simulink model "RealLifeTrainModel"  (R2024a)
settings: Solver=ode1  StartTime=0.0  StopTime=Inf  FixedStep=0.001  RelTol=1e-3
PostLoadFcn:
  | , if any(exist('dsrtsu_mdlpostloadfcn', 'file') ~= 0), dsrtsu_mdlpostloadfcn('Execute', bdroot); end,
InitFcn:
  | , if any(exist('rtifpga_mdlclblib', 'file') ~= 0), rtifpga_mdlclblib('Init', bdroot); end,
undefined symbols (not defined in the file): DiscIntNeverNeededParam
libraries: deeplib x29, svdutilitieslib x28, simulink x8, eeGeneralControl x8, rti1202lib_adc_class1 x6, rti1202serlib x5, spsEdgeDetectorLib x5, rtiemclib x2, rti1202lib_dac_class1 x1
(part 8 of 8)

== matlab function RealLifeTrainModel/ContractionMetricFilterSystem1/MATLAB Function ==
  data: x input; u_filtered output; ref input; u_nom input; dt input; task_dim input; row_major input; td_is_zero_based input; eps_pd input; use_A_transpose input; lambda_val input; last_ixv input; flag_start input; Kp input; Ki input; ref_denorm input; Dref_denorm input; integral_erro input; cert_val output; is_active output; a_val output; b_val output; du_out output; M_curr_out output; Mdot_out output; erro output; u_nom_teste output; A_m output; B_m output; K_m output; k1 input; k2 input; k3 input; dkp input; dki input; controller input
function [u_filtered, cert_val, is_active, a_val, b_val, du_out, M_curr_out, Mdot_out,erro,u_nom_teste,A_m,B_m,K_m] = ...
    qp_filter_projected_deltaU_getM( ...
        x, ref, u_nom, ...
        dt, task_dim, ...
        row_major, td_is_zero_based, eps_pd, use_A_transpose, lambda_val, ...
        last_ixv, flag_start, Kp, Ki, ref_denorm, Dref_denorm,integral_erro,k1,k2,k3,dkp,dki,controller) %#codegen

max_Fload =  569.629505294963
min_Fload = -610.339671010468

% Closed-form QP:  min 0.5*||Δu||^2  s.t. a'*Δu <= b,   u_filt = u_nom + Δu
% Uses your get_M(x) to build M(x) internally (no M_* inputs).
% A,B from FD on get_model([x;u]), K from FD on your policy(...).

% -------- defaults / casts (codegen-safe) --------
if nargin < 6  || isempty(row_major),        row_major        = true;  end %#ok<NASGU> % kept for API compat; get_M already fixes orientation
if nargin < 7  || isempty(td_is_zero_based), td_is_zero_based = true;  end
if nargin < 8  || isempty(eps_pd),           eps_pd           = single(1e-3); end
if nargin < 9  || isempty(use_A_transpose),  use_A_transpose  = false; end

tdZeroBased = (td_is_zero_based ~= 0);
useAT       = (use_A_transpose  ~= 0);

dt          = cast(dt,          'single');
eps_pd      = cast(eps_pd,      'single');
lambda_val  = cast(lambda_val,  'single');
Kp          = cast(Kp,          'single');
Ki          = cast(Ki,          'single');
ref_denorm  = cast(ref_denorm,  'single');
Dref_denorm = cast(Dref_denorm, 'single');
last_ixv    = cast(last_ixv,    'single');
flag_start  = cast(flag_start,  'single');

% -------- sizes / shapes --------
n   = int32(8);                 % state dim
m   = int32(1);                 % scalar control
x_m = reshape(x, [], 1);        % (n x 1), normalized [0,1]

% -------- Metric from your network --------
M_curr = cast(get_M(x_m), 'single');    % (8x8) SPD already
M_curr_out = M_curr;                    % expose for debug

% -------- Compute Mdot --------
persistent have_prev M_prev
if isempty(have_prev)
    have_prev = false;
    M_prev    = zeros(8,8,'single');
end

if flag_start ~= 0
    % reset at episode start
    have_prev = false;
end


M_dot = (M_curr - M_prev) ./ dt;    % time FD


% update persistent for next call
M_prev    = M_curr;
have_prev = true;

Mdot_out = M_dot;    % expose for debug

%policy(normdata,last_ixv,flag_start,ref_denorm,Kp,Ki,Dref_denorm,integral)
u_nom_teste = 2*policy_nominal_(x_m,ref,last_ixv,flag_start,Kp,Ki,ref_denorm,Dref_denorm,integral_erro,dkp,dki,controller) - 1

% -------- Linearize model: A = ∂f/∂x, B = ∂f/∂u --------
[A_m, B_m] = linearize_model_fd_(x_m, u_nom, n);

% -------- K from your policy (FD) --------

K_m = policy_jacobian_fd_(x_m, ref, last_ixv, flag_start, Kp, Ki, ref_denorm, Dref_denorm, n,integral_erro,dkp,dki,controller); % (1 x n)

% -------- ABK (+ optional Aᵀ) --------
A_use = A_m; if useAT, A_use = A_m.'; end
ABK   = A_use + B_m * K_m;     % (n x n)

% -------- Contraction matrix --------
symPart = M_curr * ABK;
symPart = symPart + symPart.'; 
C = M_dot + symPart + (2 * lambda_val) * M_curr;

% -------- contracting direction v --------
td = int32(task_dim); if tdZeroBased, td = td + 1; end
td = max(1, min(td, n));
v = zeros(n,1,'single');
v(td,1) = cast(x_m(td,1) - cast(ref,'like',x_m), 'single');

% -------- certificate & halfspace --------
cert_val = cast(v' * C * v, 'like', u_nom);      % scalar
a_row    = 2 * (v' * (M_curr * B_m));            % (1 x m)
e = ref - x(3)
b_val    = cast(-(v' * C * v), 'like', u_nom) - (k2 + k3*abs(e));   % scalar

% -------- closed-form projection in Δu-space --------
a_col  = cast(a_row.', 'like', u_nom);           % (m x 1)
anorm2 = max(cast(1e-12, 'like', u_nom), sum(a_col .* a_col));

if b_val >= 0
    du = zeros(m, 1, 'like', u_nom); active = 0;
else
    du = (b_val / anorm2) * a_col;   active = 1;
end

% elementwise clip Δu
du = min(max(du, -eps_pd), eps_pd);

u_filtered = u_nom + du + k1*(e);
is_active  = double(active);
a_val      = a_col;
du_out     = du;

force = x(3)*(max_Fload - min_Fload) + min_Fload

erro = ref_denorm - force
end

% ====================== helpers (codegen-safe) ======================

function y = clip01_(z)
% clamp to [0,1] (single, vector/scalar)
y = min(max(cast(z,'single'), cast(0,'single')), cast(1,'single'));
end

function [A_m, B_m] = linearize_model_fd_(x, u, n)
% Central FD on your ONNX-backed model get_model([x;u])
x = cast(x, 'single'); u = cast(u, 'single');
A_m = zeros(n, n, 'single');
B_m = zeros(n, 1, 'single');

eps_x = cast(1e-4, 'single');
eps_u = cast(1e-3, 'single');

xm = clip01_(x);
f = f_model_(x, u);

% A: ∂f/∂x
for i = 1:n
    dx = zeros(n,1,'single'); dx(i) = eps_x;
    xp = (x + dx);

    fp = f_model_(xp, u);

    A_m(:, i) = (fp - f) ./ (eps_x);
end

% B: ∂f/∂u
up = (u + eps_u);
ul = (u - eps_u);
xm = clip01_(x);
fp = f_model_(x, up);
fl = f_model_(x, ul);

B_m(:, 1) = (fp - f) ./ (eps_u);
end

function f = f_model_(x, u)
% Evaluate learned dynamics at (x,u); get_model expects 9x1 input [x; u]
xu = [cast(x,'single'); cast(u,'single')];
f  = cast(get_model(xu), 'single');   % (8x1)
end

function K = policy_jacobian_fd_(x, ref, last_ixv, flag_start, Kp, Ki, ref_denorm, Dref_denorm, n,integral,dkp,dki,controller)
% Central FD of your policy π(x, ref) using your provided function
K = zeros(1, n, 'single');
eps_x = cast(1e-3, 'single');
x_ = (x);
u = policy_nominal_(x_, ref, last_ixv, flag_start, Kp, Ki, ref_denorm, Dref_denorm,integral,dkp,dki,controller);

for i = 1:n
    dx = zeros(n,1,'single'); dx(i) = eps_x;
    xp = (x + dx);

    up = policy_nominal_(xp, ref, last_ixv, flag_start, Kp, Ki, ref_denorm, Dref_denorm,integral,dkp,dki,controller);

    K(1,i) = (up - u) ./ (eps_x);
end
end

function u = policy_nominal_(x, ref, last_ixv, flag_start, Kp, Ki, ref_denorm, Dref_denorm,integral,dkp,dki,controller)
% Thin wrapper to your policy(normdata,last_ixv,flag_start,ref_denorm,Kp,Ki,Dref_denorm)
normdata = [cast(x,'single'); cast(ref,'single')];  % 9x1, normalized
u = cast(policy(normdata, last_ixv, flag_start, ref_denorm, Kp, Ki, Dref_denorm,integral,dkp,dki,controller), 'single');
end


function y = get_model(x)
%#codegen
% x: 9x1 normalized in [0,1]
% y: 8x1 single, normalized to [0,1]
% y = y1 + (y2.^2) * u_scalar, then re-scale to [0,1]

% ---- normalize / split inputs ----
x_single = single(x(:));           % 9x1
x_scaled = 2*x_single - 1;         % [-1, 1]
feat     = x_scaled(1:8);          % 8x1
u_scalar = x_scaled(9);            % scalar

% ---- two pure-C forwards using saved weights ----
y1 = model_forward_m1(x_scaled);       % 8x1


% ---- combine and clamp ----

y  = 0.5 * y1 + 0.5;                % back to [0,1]
end


function M = get_M(x)
%#codegen
% x: 8x1 normalized in [0,1]
% M: 8x8 SPD single

x8  = single(x(:));                % 8x1

% metric net: 2-FC (64 outputs) → reshape to 8x8
v64 = metric_forward_2fc(x8);      % 64x1

n    = int32(8);
Mraw = reshape(v64, [n, n]).';                          % row-major → col-major
M    = (Mraw.' * Mraw) + single(1e-3) * eye(n,'single'); % SPD
end


% ==================== helpers (pure C, RTI-safe) ====================

function y = model_forward_m1(x8)
%#codegen
% 3-FC with ReLU after first two; outputs 8x1
persistent W1 b1 W2 b2 W3 b3 init
if isempty(init)
    S  = coder.load(coder.const('C:\Users\ic2d\Documents\GitHub\dSpace_Controllers_legged\model_smaller_weights.mat'));
    W1 = single(S.W1);  b1 = single(S.b1);   % [64x8],  [64x1]
    W2 = single(S.W2);  b2 = single(S.b2);   % [64x64], [64x1]
    W3 = single(S.W3);  b3 = single(S.b3);   % [8x64],  [8x1]
    init = true;
end
x8 = single(x8(:));
z1 = W1 * x8 + b1;   a1 = max(z1, single(0));   % ReLU
z2 = W2 * a1 + b2;   a2 = max(z2, single(0));   % ReLU
y  = W3 * a2 + b3;                              % 8x1
end

function y = model_forward_m2(x8)
%#codegen
% 3-FC with ReLU after first two; outputs 8x1
persistent W1 b1 W2 b2 W3 b3 init
if isempty(init)
    S  = coder.load(coder.const('C:\Users\ic2d\Documents\GitHub\dSpace_Controllers_legged\model_2_weights.mat'));
    W1 = single(S.W1);  b1 = single(S.b1);   % [64x8],  [64x1]
    W2 = single(S.W2);  b2 = single(S.b2);   % [64x64], [64x1]
    W3 = single(S.W3);  b3 = single(S.b3);   % [8x64],  [8x1]
    init = true;
end
x8 = single(x8(:));
z1 = W1 * x8 + b1;   a1 = max(z1, single(0));   % ReLU
z2 = W2 * a1 + b2;   a2 = max(z2, single(0));   % ReLU
y  = W3 * a2 + b3;                              % 8x1
end

function y64 = metric_forward_2fc(x8)
%#codegen
% 2-FC with ReLU after first; outputs 64x1
persistent W1 b1 W2 b2 init
if isempty(init)
    S  = coder.load(coder.const('C:\Users\ic2d\Documents\GitHub\dSpace_Controllers_legged\metric_new_weights.mat'));
    W1 = single(S.W1);  b1 = single(S.b1);   % [64x8],  [64x1]
    W2 = single(S.W2);  b2 = single(S.b2);   % [64x64], [64x1]
    init = true;
end
x8  = single(x8(:));
z1  = W1 * x8 + b1;                 % [64x1]
a1  = max(z1, single(0));           % ReLU
y64 = W2 * a1 + b2;                 % [64x1]
end


function y = policy(normdata,last_ixv,flag_start,ref_denorm,Kp,Ki,Dref_denorm,integral,dkp,dki,controller)

data = denorm(normdata)

y = FL(last_ixv,flag_start,data, Kp,Ki,Dref_denorm,ref_denorm,integral,dkp,dki,controller);

end


function y = denorm(u)
    max_Fload =  569.629505294963
    min_Fload = -610.339671010468
    
    max_Fhyd = 729.261146885585
    min_Fhyd = -777.489547410502
    
    max_DFload = 123011.265014651
    min_DFload = -142353.177843906
    
    max_DFhyd = 219994.429294316
    min_DFhyd = -270882.694509076
    
    max_Pa = 12037835.3221229
    min_Pa = 1849925.22965178
    
    max_Pb = 14831789.6053956
    min_Pb = 2808786.27887814
    
    max_x = 0.082368752
    min_x = 0.01990812
    
    max_Dx = 0.682789396628826
    min_Dx = -0.578996654196926
    
    out = [1,1,1,1,1,1,1,1,1]
    
    out(1) = (u(1))*(max_Fhyd - min_Fhyd) + min_Fhyd;
    
    out(2) = (u(2))*(max_DFhyd - min_DFhyd) + min_DFhyd;
    
    out(3) = (u(3))*(max_Fload - min_Fload) + min_Fload;
    
    out(4) = (u(4))*(max_DFload - min_DFload) + min_DFload;
    
    out(5) = (u(5))*(max_Pa - min_Pa) + min_Pa;
    
    out(6) = (u(6))*(max_Pb - min_Pb) + min_Pb;
    
    out(7) = (u(7))*(max_x - min_x) + min_x;
    
    out(8) = (u(8))*(max_Dx - min_Dx) + min_Dx;
    
    out(9) = (u(9))*(max_Fload - min_Fload) + min_Fload;
    
    
    y = out;
end

function y = FL(ixv,flag_start,data_denorm,Kp,Ki,Dref_denorm,Ref_denorm,integral,dkp,dki,controller)
    Pn = 7000000
    Qn = 10/60000
    Un = 0.05
    Be = 1.31E+9
    c1 = 0.8
    c2 = 1
    alfa = 0.609
    Vpl = 0.00121
    Ps = 16000000
    Pt = 0
    L_cyl = 0.08
    Aa = 0.000201
    
    if flag_start == 1
        data = data_denorm
        Pa = data(5)
        Pb = data(6)
        xp = data(7)
        xpd = data(8)
    
        Kv = Qn/(Un*sqrt(Pn/2));
        
        Va = Vpl + Aa*xp;
        Vb = Vpl + (L_cyl - xp)*alfa*Aa;
    
        if(ixv >= 0)
            g = Be*Aa*Kv*( sign(Ps-Pa)*sqrt(abs(Ps-Pa))/Va + alfa*sign(Pb-Pt)*sqrt(abs(Pb-Pt))/Vb);
        else
            g = Be*Aa*Kv*( sign(Pa-Pt)*sqrt(abs(Pa-Pt))/Va + alfa*sign(Ps-Pb)*sqrt(abs(Ps-Pb))/Vb);
        end
        
        %g1 = Be*Aa*Kv*( sign(Ps-Pa)*sqrt(abs(Ps-Pa))/Va + alfa*sign(Pb-Pt)*sqrt(abs(Pb-Pt))/Vb);
        %g2 = Be*Aa*Kv*( sign(Pa-Pt)*sqrt(abs(Pa-Pt))/Va + alfa*sign(Ps-Pb)*sqrt(abs(Ps-Pb))/Vb);
        %g = (g1 + g2)/2;
    
        f = -Be*Aa^2*(((alfa)^2)/Vb + 1/Va)*xpd;
        
        g = c2*g;
        f = c1*f;

        self_max_d = 0.0005
        self_min_d = -0.0005
        self_mean_d = self_max_d/2 + self_min_d/2
    
        self_max_c1 = 1.0 + 0.05
        self_min_c1 = 1.0 - 0.05
        self_mean_c1 = self_max_c1/2 + self_min_c1/2
    
        self_max_c2 = 1.0 + 0.05
        self_min_c2 = 1.0 - 0.05
        self_mean_c2 = sqrt(self_max_c2*self_min_c2)
    
        self_eta = 1
        beta = sqrt(self_max_c2/self_min_c2)

        error = Ref_denorm - data(3);
        integral_error = integral;

        psi = 600;
        dref = Dref_denorm;
        dx = xpd;
        h = f;
        dist = 0;
        kp = Kp;
        ki = Ki;
    
        s = -kp*error -ki*integral_error
    
        u = kp*(-self_mean_c1*h - g*self_mean_d + dref) + dkp*error + ki*error + dki*integral_error
        k = abs(beta - 1)*abs(u) + beta*kp*(self_max_c1 - self_mean_c1)*abs(h) + beta*kp*(self_max_d - self_mean_d)*abs(g) + self_eta*beta
        
        sat_ = single(0)
    
        if(abs(s/psi) <= 1)
            sat_ = s/psi;
        
        else
            if(s >= 0)
                sat_ = single(1); 
            
            elseif(s < 0)
                sat_ = single(-1); 
            end
        end
        gain_vc = 0.032

        selector = controller;

        if(selector == 0)
            y = (u - k*sat_)/(self_mean_c2*kp*g)
        elseif(selector == 1)
            y = kp*error + ki*integral_error + gain_vc*dx
        else
            y = (kp*error + ki*integral_error + dref - h)/g - dist
        end
        
    
        y = y/0.05;
        y = y/2 + 0.5

 

    else
        y = single(0)
    end
end

== matlab function RealLifeTrainModel/ContractionMetricFilterSystem1/MATLAB Function1 ==
  data: u input; KP output; Kp_s input; Ki_s input; KI output
function [KP,KI] = fcn(u,Kp_s,Ki_s)

persistent kp_hold ki_hold hold_count

if(u == 1)
    if isempty(hold_count)
        % First-time init
        kp_hold    = 15 + 80 * rand();   % KP in [15, 95]
        ki_hold    = 0;                   % match your original: KI forced to 0
        hold_count = 10;                  % hold for 10 steps
    end
    
    % Re-draw when the 10-step window expires OR when u==1 (manual reset)
    if (hold_count <= 0) || (u == 1)
        kp_hold    = 15 + 80 * rand();   % KP in [15, 95]
        ki_hold    = 0;                   % set KI to 0 (change here if you want it random)
        hold_count = 10;
    end
    
    % Output the held values
    KP = kp_hold;
    KI = ki_hold;
    
    % Consume one time step of the hold window
    hold_count = hold_count - 1;

else
    KP = Kp_s
    KI = Ki_s
end

== matlab function RealLifeTrainModel/ContractionMetricFilterSystem1/NormalizeMetric_1 ==
  data: u input; y output
function y = fcn(u)

max_Fload =  569.629505294963
min_Fload = -610.339671010468

max_Fhyd = 729.261146885585
min_Fhyd = -777.489547410502

max_DFload = 123011.265014651
min_DFload = -142353.177843906

max_DFhyd = 219994.429294316
min_DFhyd = -270882.694509076

max_Pa = 12037835.3221229
min_Pa = 1849925.22965178

max_Pb = 14831789.6053956
min_Pb = 2808786.27887814

max_x = 0.082368752
min_x = 0.01990812

max_Dx = 0.682789396628826
min_Dx = -0.578996654196926

out = [1,1,1,1,1,1,1,1]

out(1) = (u(1) - min_Fhyd)/(max_Fhyd - min_Fhyd);
out(2) = (u(2) - min_DFhyd)/(max_DFhyd - min_DFhyd);
out(3) = (u(3) - min_Fload)/(max_Fload - min_Fload);
out(4) = (u(4) - min_DFload)/(max_DFload - min_DFload);
out(5) = (u(5) - min_Pa)/(max_Pa - min_Pa);
out(6) = (u(6) - min_Pb)/(max_Pb - min_Pb);
out(7) = (u(7) - min_x)/(max_x - min_x);
out(8) = (u(8) - min_Dx)/(max_Dx - min_Dx);



y = out;

== matlab function RealLifeTrainModel/ContractionMetricFilterSystem1/NormalizeMetric_2 ==
  data: u input; y output
function y = fcn(u)

max_Fload =  569.629505294963
min_Fload = -610.339671010468

max_Fhyd = 729.261146885585
min_Fhyd = -777.489547410502

max_DFload = 123011.265014651
min_DFload = -142353.177843906

max_DFhyd = 219994.429294316
min_DFhyd = -270882.694509076

max_Pa = 12037835.3221229
min_Pa = 1849925.22965178

max_Pb = 14831789.6053956
min_Pb = 2808786.27887814

max_x = 0.082368752
min_x = 0.01990812

max_Dx = 0.682789396628826
min_Dx = -0.578996654196926

out = [1]


out(1) = (u(1) - min_Fload)/(max_Fload - min_Fload);




y = out;

== matlab function RealLifeTrainModel/ContractionMetricFilterSystem1/Normalize_Policy ==
  data: u input; y output
function y = fcn(u)

max_Fload =  569.629505294963
min_Fload = -610.339671010468

max_Fhyd = 729.261146885585
min_Fhyd = -777.489547410502

max_DFload = 123011.265014651
min_DFload = -142353.177843906

max_DFhyd = 219994.429294316
min_DFhyd = -270882.694509076

max_Pa = 12037835.3221229
min_Pa = 1849925.22965178

max_Pb = 14831789.6053956
min_Pb = 2808786.27887814

max_x = 0.082368752
min_x = 0.01990812

max_Dx = 0.682789396628826
min_Dx = -0.578996654196926

out = [1,1,1,1,1,1,1,1,1]

out(1) = (u(1) - min_Fhyd)/(max_Fhyd - min_Fhyd);
out(2) = (u(2) - min_DFhyd)/(max_DFhyd - min_DFhyd);
out(3) = (u(3) - min_Fload)/(max_Fload - min_Fload);
out(4) = (u(4) - min_DFload)/(max_DFload - min_DFload);
out(5) = (u(5) - min_Pa)/(max_Pa - min_Pa);
out(6) = (u(6) - min_Pb)/(max_Pb - min_Pb);
out(7) = (u(7) - min_x)/(max_x - min_x);
out(8) = (u(8) - min_Dx)/(max_Dx - min_Dx);

out(9) = (u(9) - min_Fload)/(max_Fload - min_Fload);


y = out;

== matlab function RealLifeTrainModel/ContractionMetricFilterSystem1/Policy_SS/Denormalize_Policy ==
  data: u input; y output
function y = fcn(u)

max_Fload =  569.629505294963
min_Fload = -610.339671010468

max_Fhyd = 729.261146885585
min_Fhyd = -777.489547410502

max_DFload = 123011.265014651
min_DFload = -142353.177843906

max_DFhyd = 219994.429294316
min_DFhyd = -270882.694509076

max_Pa = 12037835.3221229
min_Pa = 1849925.22965178

max_Pb = 14831789.6053956
min_Pb = 2808786.27887814

max_x = 0.082368752
min_x = 0.01990812

max_Dx = 0.682789396628826
min_Dx = -0.578996654196926

out = [1,1,1,1,1,1,1,1,1]

out(1) = (u(1))*(max_Fhyd - min_Fhyd) + min_Fhyd;

out(2) = (u(2))*(max_DFhyd - min_DFhyd) + min_DFhyd;

out(3) = (u(3))*(max_Fload - min_Fload) + min_Fload;

out(4) = (u(4))*(max_DFload - min_DFload) + min_DFload;

out(5) = (u(5))*(max_Pa - min_Pa) + min_Pa;

out(6) = (u(6))*(max_Pb - min_Pb) + min_Pb;

out(7) = (u(7))*(max_x - min_x) + min_x;

out(8) = (u(8))*(max_Dx - min_Dx) + min_Dx;

out(9) = (u(9))*(max_Fload - min_Fload) + min_Fload;


y = out;

== matlab function RealLifeTrainModel/ContractionMetricFilterSystem1/Policy_SS/FLcontroller1 ==
  data: kp input; y output; ki input; error input; integral_error input; dref input; h input; g input; dkp input; dki input; flag_start input; psi input; dx input; gain_vc input; selector input; slide_margin input; dist input; slide_dist_max input; slide_dist_min input; teste output; leak input
function [y,teste] = fcn(kp, ki, error, integral_error,dref,h,g,dkp,dki,flag_start,psi,dx,gain_vc,selector,slide_margin,dist,slide_dist_max,slide_dist_min,leak)

if flag_start == 1
    self_max_d = slide_dist_max
    self_min_d = slide_dist_min
    self_mean_d = self_max_d/2 + self_min_d/2

    self_max_c1 = 1.0 + slide_margin
    self_min_c1 = 1.0 - slide_margin
    self_mean_c1 = self_max_c1/2 + self_min_c1/2

    self_max_c2 = 1.0 + slide_margin
    self_min_c2 = 1.0 - slide_margin
    self_mean_c2 = sqrt(self_max_c2*self_min_c2)

    self_eta = 1
    beta = sqrt(self_max_c2/self_min_c2)


    s = -kp*error -ki*integral_error

    u = kp*(-self_mean_c1*h -self_mean_c2*leak - g*self_mean_d + dref) + dkp*error + ki*error + dki*integral_error
    k = abs(beta - 1)*abs(u) + beta*kp*(self_max_c1 - self_mean_c1)*abs(h) + beta*kp*(self_max_c2 - self_mean_c2)*abs(leak) + beta*kp*(self_max_d - self_mean_d)*abs(g) + self_eta*beta
    
    sat_ = 0

    if(abs(s/psi) <= 1)
        sat_ = s/psi;
    
    else
        if(s >= 0)
            sat_ = 1; 
        
        elseif(s < 0)
            sat_ = -1; 
        end
    end

    teste = 0
    teste = ((-h/g)/dx)
    if(selector == 0)
        y = (u - k*sat_)/(self_mean_c2*kp*g)
    elseif(selector == 1)
    
        y = kp*error + ki*integral_error + gain_vc*dx
    else
        y = (kp*error + ki*integral_error + dref - h - leak)/g - dist
    end
    
else 
    teste = 0
    y = 1;
end

== matlab function RealLifeTrainModel/ContractionMetricFilterSystem1/Policy_SS/FunctionCalculateHydModel1 ==
  data: ixv input; f output; Pn input; Qn input; Un input; Vpl input; Ps input; Pt input; L_cyl input; Aa input; alfa input; c1 input; c2 input; Be input; flag_start input; data input; g output; force output; xpd output
function [f,g,force,xpd] = fcn(ixv,Pn,Qn,Un,Vpl,Ps,Pt,L_cyl,Aa,alfa,c1,c2,Be,flag_start,data)
force = 0
xpd =0
if flag_start == 1
    Pa = data(5)
    Pb = data(6)
    xp = data(7)
    xpd = data(8)
    force = data(3)

    Kv = Qn/(Un*sqrt(Pn/2));
    
    Va = Vpl + Aa*xp;
    Vb = Vpl + (L_cyl - xp)*alfa*Aa;

    if(ixv >= 0)
        g = Be*Aa*Kv*( sign(Ps-Pa)*sqrt(abs(Ps-Pa))/Va + alfa*sign(Pb-Pt)*sqrt(abs(Pb-Pt))/Vb);
    else
        g = Be*Aa*Kv*( sign(Pa-Pt)*sqrt(abs(Pa-Pt))/Va + alfa*sign(Ps-Pb)*sqrt(abs(Ps-Pb))/Vb);
    end
    
    %g1 = Be*Aa*Kv*( sign(Ps-Pa)*sqrt(abs(Ps-Pa))/Va + alfa*sign(Pb-Pt)*sqrt(abs(Pb-Pt))/Vb);
    %g2 = Be*Aa*Kv*( sign(Pa-Pt)*sqrt(abs(Pa-Pt))/Va + alfa*sign(Ps-Pb)*sqrt(abs(Ps-Pb))/Vb);
    %g = (g1 + g2)/2;

    f = -Be*Aa^2*(((alfa)^2)/Vb + 1/Va)*xpd;
    
    g = c2*g;
    f = c1*f;
    
else
    f = 1;
    g = 1;
end

== matlab function RealLifeTrainModel/ContractionMetricFilterSystem1/Policy_SS/Policy ==
  data: u input; y output
function y = fcn(u)

y = (u)/2 + 0.5;

== matlab function RealLifeTrainModel/ContractionMetricFilterSystem1/Renormalize ==
  data: u input; y output
function y = fcn(u)

y = u*2 - 1;

== matlab function RealLifeTrainModel/PolyDerivativeSubSystem4/MATLAB Function ==
  data: k input; dx output; Ts input; ddx output; dddx output
function [dx,ddx,dddx] = poly_derivative(k,Ts)
    T =0 ;
    x = [k(1),k(2),k(3),k(4),k(5),k(6),k(7),k(8),k(9),k(10),k(11),k(12),k(13),k(14),k(15),k(16),k(17),k(18),k(19),k(20)];
    t = [T,T-1*Ts,T-2*Ts,T-3*Ts,T-4*Ts,T-5*Ts,T-6*Ts,T-7*Ts,T-8*Ts,T-9*Ts,T-10*Ts,T-11*Ts,T-12*Ts,T-13*Ts,T-14*Ts,T-15*Ts,T-16*Ts,T-17*Ts,T-18*Ts,T-19*Ts];

    p = polyfit(t, x, 3);    

    dp = polyder(p);         % derivative
    ddp = polyder(dp);
    dddp = polyder(ddp)
    
    dx = polyval(dp, T);     % evaluate at current time
    ddx = polyval(ddp, T)
    dddx = polyval(dddp, T)
end

== matlab function RealLifeTrainModel/ContractionMetricFilterSystem3/CalcK/IndidualGrad1/MATLAB Function2 ==
  data: u input; y output; pos input
function y = fcn(u,pos)

a = [0,0,0,0,0,0,0,0,0]

a(pos) = u

y = a;

== matlab function RealLifeTrainModel/ContractionMetricFilterSystem3/CalcK/IndidualGrad1/MATLAB Function5 ==
  data: u1 input; y output; u2 input; const input
function y = fcn(u1,u2,const)

y = (u1 - u2)/(const);

== matlab function RealLifeTrainModel/ContractionMetricFilterSystem3/CalcK/IndidualGrad1/Policy_SS1/Denormalize_Policy ==
  data: u input; y output
function y = fcn(u)

max_Fload =  569.629505294963
min_Fload = -610.339671010468

max_Fhyd = 729.261146885585
min_Fhyd = -777.489547410502

max_DFload = 123011.265014651
min_DFload = -142353.177843906

max_DFhyd = 219994.429294316
min_DFhyd = -270882.694509076

max_Pa = 12037835.3221229
min_Pa = 1849925.22965178

max_Pb = 14831789.6053956
min_Pb = 2808786.27887814

max_x = 0.082368752
min_x = 0.01990812

max_Dx = 0.682789396628826
min_Dx = -0.578996654196926

out = [1,1,1,1,1,1,1,1,1]

out(1) = (u(1))*(max_Fhyd - min_Fhyd) + min_Fhyd;

out(2) = (u(2))*(max_DFhyd - min_DFhyd) + min_DFhyd;

out(3) = (u(3))*(max_Fload - min_Fload) + min_Fload;

out(4) = (u(4))*(max_DFload - min_DFload) + min_DFload;

out(5) = (u(5))*(max_Pa - min_Pa) + min_Pa;

out(6) = (u(6))*(max_Pb - min_Pb) + min_Pb;

out(7) = (u(7))*(max_x - min_x) + min_x;

out(8) = (u(8))*(max_Dx - min_Dx) + min_Dx;

out(9) = (u(9))*(max_Fload - min_Fload) + min_Fload;


y = out;

== matlab function RealLifeTrainModel/ContractionMetricFilterSystem3/CalcK/IndidualGrad1/Policy_SS1/FLcontroller1 ==
  data: pid input; y output; f input; g input; dFref input; d input; flag_start input
function y = fcn(pid,f,g,dFref,d,flag_start)

if flag_start == 1
    y = (dFref + pid - f)/g - d;
else 
    y = 1;
end

== matlab function RealLifeTrainModel/ContractionMetricFilterSystem3/CalcK/IndidualGrad1/Policy_SS1/FunctionCalculateHydModel1 ==
  data: ixv input; f output; Pn input; Qn input; Un input; Vpl input; Ps input; Pt input; L_cyl input; Aa input; alfa input; c1 input; c2 input; Be input; flag_start input; data input; g output; force output
function [f,g,force] = fcn(ixv,Pn,Qn,Un,Vpl,Ps,Pt,L_cyl,Aa,alfa,c1,c2,Be,flag_start,data)
force = 0
if flag_start == 1
    Pa = data(5)
    Pb = data(6)
    xp = data(7)
    xpd = data(8)
    force = data(3)

    Kv = Qn/(Un*sqrt(Pn/2));
    
    Va = Vpl + Aa*xp;
    Vb = Vpl + (L_cyl - xp)*alfa*Aa;

    if(ixv >= 0)
        g = Be*Aa*Kv*( sign(Ps-Pa)*sqrt(abs(Ps-Pa))/Va + alfa*sign(Pb-Pt)*sqrt(abs(Pb-Pt))/Vb);
    else
        g = Be*Aa*Kv*( sign(Pa-Pt)*sqrt(abs(Pa-Pt))/Va + alfa*sign(Ps-Pb)*sqrt(abs(Ps-Pb))/Vb);
    end
    
    %g1 = Be*Aa*Kv*( sign(Ps-Pa)*sqrt(abs(Ps-Pa))/Va + alfa*sign(Pb-Pt)*sqrt(abs(Pb-Pt))/Vb);
    %g2 = Be*Aa*Kv*( sign(Pa-Pt)*sqrt(abs(Pa-Pt))/Va + alfa*sign(Ps-Pb)*sqrt(abs(Ps-Pb))/Vb);
    %g = (g1 + g2)/2;

    f = -Be*Aa^2*(((alfa)^2)/Vb + 1/Va)*xpd;
    
    g = c2*g;
    f = c1*f;
    
else
    f = 1;
    g = 1;
end
